simulink model "multi_ca_sim_1"  (R2020a)
settings: Solver=FixedStepAuto  StartTime=0.0  StopTime=23  FixedStep=0.01  MinStep=0.01  RelTol=1e-3
values from neighbouring files (symbols this model uses):
  ar_max = beta^2*omega/gamma/pi*0.999    (= 2.172825)    [SimulationSetup.m]
  beta = pi/tau_r    (= 3.14159265359)    [SimulationSetup.m]
  gamma = tau_r*beta + pi    (= 6.28318530718)    [SimulationSetup.m]
  Gamma = 10    [SimulationSetup.m]
  k = (gamma/beta)^2*(vo_max*psio_max) +0.1    (= 0.235)    [SimulationSetup.m]
  k_1 = 0.2    [SimulationSetup.m]
  k_2 = gamma^2/beta    (= 12.5663706144)    [SimulationSetup.m]
  k_delta = 1    [SimulationSetup.m]
  omega = r + (vr_max + vo_max)*pi/beta +0.1    (= 4.35)    [SimulationSetup.m]
  r = 2.0    (= 2)    [SimulationSetup.m]
  theta_0_1 = 0    [SimulationSetup.m]
  theta_0_2 = 0    [SimulationSetup.m]
  theta_0_3 = 0    [SimulationSetup.m]
  theta_a = pi/4    (= 0.785398163397)    [SimulationSetup.m]
  u_ca_max = 10    [SimulationSetup.m]
  u_tr_max = min(beta,beta^2*omega/(vr_max*gamma))    [SimulationSetup.m]
  vo_max = 0.75    [SimulationSetup.m]
  vr_max = 1.5    [SimulationSetup.m]
  vr_min = 1.0    (= 1)    [SimulationSetup.m]
  x_F_0_1 = -6    [SimulationSetup.m]
  x_F_0_2 = -4    [SimulationSetup.m]
  x_F_0_3 = -5    [SimulationSetup.m]
  y_F_0_1 = 0    [SimulationSetup.m]
  y_F_0_2 = -2    [SimulationSetup.m]
  y_F_0_3 = -4    [SimulationSetup.m]
libraries: cstblocks x3, dspmathops x3
(part 2 of 2)

== matlab function multi_ca_sim_1/MATLAB Function1 ==
  data: rho output; pos_vr input; lambda output; pos_obs input; psi_r input; psi_o input; vo input; vr input; dot_lambda output
function [rho, lambda, dot_lambda] = fcn(pos_vr, pos_obs, psi_r, psi_o, vo, vr)

lambda_vector = pos_obs-pos_vr;
rho = norm(lambda_vector,2);
lambda = atan2(lambda_vector(2), lambda_vector(1) );
dot_lambda = 1/rho*(vo*sin(psi_o - lambda) - vr*sin(psi_r - lambda));

== matlab function multi_ca_sim_1/vehicle2/MATLAB Function ==
  data: u input; y output; tan output
function [y,tan] = fcn(u)
theta = u/(1.5*1.5*4*pi);
y = [cos(theta) -sin(theta); sin(theta) cos(theta)]*[1.5*1.5*4*pi; 0];%*[5+6*pi*sin(pi/4)-6*pi*sin(1.2*pi/4)-0.5 15+6*pi*cos(pi/4)-6*pi*cos(1.2*pi/4)]';
tan = [-y(2); y(1)];

== matlab function multi_ca_sim_1/vehicle2/MATLAB Function1 ==
  data: u input; y output
function y = fcn(u)
theta = u/(1.5*1.5*4*pi);
y = [cos(theta) -sin(theta); sin(theta) cos(theta)]*[1.5*1.5*4*pi; 0];%*[5+6*pi*sin(pi/4)-6*pi*sin(1.2*pi/4)-0.5 15+6*pi*cos(pi/4)-6*pi*cos(1.2*pi/4)]';

== matlab function multi_ca_sim_1/vehicle2/vehicle 1 ==
  data: speed_profile output; speed_target output; v_d_xi output; kappa output; t input; xi input; xi_dot input
function [speed_profile, speed_target, v_d_xi, kappa] = fcn(t,xi,xi_dot)
% vd=1.5;
% psi_d = t/pi/4 - pi/4;
% x_dot = 1.5*cos(psi_d);
% y_dot = 1.5*sin(psi_d);

%trajectory and speed profile
% x_dot = 1*1.5*cos(t/pi/4 - 1.2*pi/4);
% y_dot = 0.9*1.5*sin(t/pi/4 - 1.2*pi/4);
speed_profile = 1.5*1.5;

%v_d(xi)
v_d_xi=1.5*1.5;
% v_d_xi=sqrt((0.9*1.5*cos(xi/pi/4 - 1.2*pi/4))^2+(0.9*1.5*sin(xi/pi/4 - 1.2*pi/4))^2);

%speed of target
speed_target = xi_dot*1.5*1.5;

%culvature
r=1.5*1.5*4*pi;
kappa=1/r;

== matlab function multi_ca_sim_1/Time coordination/MATLAB Function5 ==
  data: xi input; Laplacian input; chi input; xi_dot output; chi_dot output
function [xi_dot, chi_dot] = fcn(xi, Laplacian, chi)
k_P=1;
k_I=0.8571; %0.95;
xi_dot=-k_P*Laplacian*xi+[1; chi(1)+0.6; chi(2)-0.2];
chi_dot=-k_I*[0 1 0; 0 0 1]*Laplacian*xi;

== matlab function multi_ca_sim_1/Subsystem/Subsystem5/Subsystem/MATLAB Function ==
  data: theta input; y output; delta input
function y = fcn(theta,delta)
if abs(theta-delta) <= 10^(-7)
    y=cos(theta);
else 
    y=(sin(theta)-sin(delta))/(theta-delta);
end

== matlab function multi_ca_sim_1/MATLAB Function2 ==
  data: tau output; rho input; loom output; rho_dot input; x4 output
function [tau, loom, x4] = fcn(rho, rho_dot)

loom = min(rho_dot/rho, 0);
if loom > -0.0001
    tau = 1000;
else
    tau = -1/loom;
end

x4 = 1/rho;

== matlab function multi_ca_sim_1/CA controller 1 ==
  data: u output; x1 input; x2 input; x3 input; x5 input; k input; r input; vr input; vo_max input; beta input; gamma input; omega input; ar input; x5 output; x2 output; x3 output; y output; alpha_1 output; alpha_2 output
function [u, x5, x2, x3,y, alpha_1, alpha_2]  = fcn(x1, x2 ,x3, x5, k, r, vr, vo_max,beta, gamma,omega, ar)


x6 = vr;

delta_t = ( pi - abs(wrapToPi_custom(x5-x2)))/(beta);

alpha_2 = -2*beta*omega*x1/(x6+vo_max);
alpha_1 = (k*x1^2 +  x6*max(0,-x3*sin(x5-x2)) -min(0, -ar*cos(x5-x2)) ) /(r + (x6 + vo_max )*delta_t);

 u =  sign_custom(wrapToPi_custom(x5-x2))*(gamma^2/beta*(x1^2  +alpha_1 ) +  alpha_2) + x3  ;
y = sign_custom(wrapToPi_custom(x5-x2));

if x1 >= 0
    u=0;
end

function y = sign_custom(x)

if x >= 0
    y = 1;
else
    y = -1;
end

function lambda = wrapTo2Pi_custom(lambda)
%wrapTo2Pi Wrap angle in radians to [0 2*pi]
%
%   lambdaWrapped = wrapTo2Pi(LAMBDA) wraps angles in LAMBDA, in radians,
%   to the interval [0 2*pi] such that zero maps to zero and 2*pi maps
%   to 2*pi. (In general, positive multiples of 2*pi map to 2*pi and
%   negative multiples of 2*pi map to zero.)
%
%   See also wrapToPi, wrapTo180, wrapTo360.

% Copyright 2007-2008 The MathWorks, Inc.

positiveInput = (lambda > 0);
lambda = mod(lambda, 2*pi);
lambda((lambda == 0) & positiveInput) = 2*pi;

function lambda = wrapToPi_custom(lambda)
%wrapToPi Wrap angle in radians to [-pi pi]
%
%   lambdaWrapped = wrapToPi(LAMBDA) wraps angles in LAMBDA, in radians,
%   to the interval [-pi pi] such that pi maps to pi and -pi maps to
%   -pi.  (In general, odd, positive multiples of pi map to pi and odd,
%   negative multiples of pi map to -pi.)
%
%   See also wrapTo2Pi, wrapTo180, wrapTo360.

% Copyright 2007-2008 The MathWorks, Inc.

q = (lambda < -pi) | (pi < lambda);
lambda(q) = wrapTo2Pi_custom(lambda(q) + pi) - pi;

== matlab function multi_ca_sim_1/Subsystem/MATLAB Function ==
  data: signal input; out output; bound1 input; bound2 input
function out = saturate(signal,bound1,bound2)
out = min(max(bound1,signal),bound2);

== matlab function multi_ca_sim_1/Time coordination/MATLAB Function3 ==
  settings: updateMethod=DISCRETE
  data: t input; y output
function y = fcn(t)

% if rem(u1,exprnd(1))==0
%     y=randi(3);
% %     if rand < 0.3
% %         y=8;
% %     else
% %         y=randi(7);
% %     end
% else
%     y=u2;

% t=u1;

rng('default')

T=[0 exprnd(1,1,60)];
i=randi(10,1,60);

% for j=1:9
%     if t>=sum(T(1:j)) && t<=sum(T(1:j+1))
%         y=i(j);
%     end
% end

        
        
if t>=sum(T(1:1)) && t<=sum(T(1:2))
    y=i(1);
elseif t>=sum(T(1:2)) && t<=sum(T(1:3))
    y=i(2);
elseif t>=sum(T(1:3)) && t<=sum(T(1:4))
    y=i(3);
elseif t>=sum(T(1:4)) && t<=sum(T(1:5))
    y=i(4);
elseif t>=sum(T(1:5)) && t<=sum(T(1:6))
    y=i(5); 
elseif t>=sum(T(1:6)) && t<=sum(T(1:7))
    y=i(6);
elseif t>=sum(T(1:7)) && t<=sum(T(1:8))
    y=i(7);
elseif t>=sum(T(1:8)) && t<=sum(T(1:9))
    y=i(8);
elseif t>=sum(T(1:9)) && t<=sum(T(1:10))
    y=i(9);
elseif t>=sum(T(1:10)) && t<=sum(T(1:11))
    y=i(10);
elseif t>=sum(T(1:11)) && t<=sum(T(1:12))
    y=i(11);
elseif t>=sum(T(1:12)) && t<=sum(T(1:13))
    y=i(12);
elseif t>=sum(T(1:13)) && t<=sum(T(1:14))
    y=i(13);
elseif t>=sum(T(1:14)) && t<=sum(T(1:15))
    y=i(14);
elseif t>=sum(T(1:15)) && t<=sum(T(1:16))
    y=i(15);
elseif t>=sum(T(1:16)) && t<=sum(T(1:17))
    y=i(16);
elseif t>=sum(T(1:17)) && t<=sum(T(1:18))
    y=i(17);
elseif t>=sum(T(1:18)) && t<=sum(T(1:19))
    y=i(18);
elseif t>=sum(T(1:19)) && t<=sum(T(1:20))
    y=i(19);
elseif t>=sum(T(1:20)) && t<=sum(T(1:21))
    y=i(20);
elseif t>=sum(T(1:21)) && t<=sum(T(1:22))
    y=i(21);
elseif t>=sum(T(1:22)) && t<=sum(T(1:23))
    y=i(22);
elseif t>=sum(T(1:23)) && t<=sum(T(1:24))
    y=i(23);
elseif t>=sum(T(1:24)) && t<=sum(T(1:25))
    y=i(24);
elseif t>=sum(T(1:25)) && t<=sum(T(1:26))
    y=i(25);
elseif t>=sum(T(1:26)) && t<=sum(T(1:27))
    y=i(26);
elseif t>=sum(T(1:27)) && t<=sum(T(1:28))
    y=i(27);
elseif t>=sum(T(1:28)) && t<=sum(T(1:29))
    y=i(28);
elseif t>=sum(T(1:29)) && t<=sum(T(1:30))
    y=i(29);
elseif t>=sum(T(1:30)) && t<=sum(T(1:31))
    y=i(30);
    elseif t>=sum(T(1:31)) && t<=sum(T(1:32))
    y=i(31);
    elseif t>=sum(T(1:32)) && t<=sum(T(1:33))
    y=i(32);
    elseif t>=sum(T(1:33)) && t<=sum(T(1:34))
    y=i(33);
    elseif t>=sum(T(1:34)) && t<=sum(T(1:35))
    y=i(34);
    elseif t>=sum(T(1:35)) && t<=sum(T(1:36))
    y=i(35);
    elseif t>=sum(T(1:36)) && t<=sum(T(1:37))
    y=i(36);
    elseif t>=sum(T(1:37)) && t<=sum(T(1:38))
    y=i(37);
    elseif t>=sum(T(1:38)) && t<=sum(T(1:39))
    y=i(38);
    elseif t>=sum(T(1:39)) && t<=sum(T(1:40))
    y=i(39);
    elseif t>=sum(T(1:40)) && t<=sum(T(1:41))
    y=i(40);
    elseif t>=sum(T(1:41)) && t<=sum(T(1:42))
    y=i(41);
    elseif t>=sum(T(1:42)) && t<=sum(T(1:43))
    y=i(42);
    elseif t>=sum(T(1:43)) && t<=sum(T(1:44))
    y=i(43);
    elseif t>=sum(T(1:44)) && t<=sum(T(1:45))
    y=i(44);
    elseif t>=sum(T(1:45)) && t<=sum(T(1:46))
    y=i(45);
    elseif t>=sum(T(1:46)) && t<=sum(T(1:47))
    y=i(46);
    elseif t>=sum(T(1:47)) && t<=sum(T(1:48))
    y=i(47);
    elseif t>=sum(T(1:48)) && t<=sum(T(1:49))
    y=i(48);
    elseif t>=sum(T(1:49)) && t<=sum(T(1:50))
    y=i(49);
    elseif t>=sum(T(1:50)) && t<=sum(T(1:51))
    y=i(50);
    elseif t>=sum(T(1:51)) && t<=sum(T(1:52))
    y=i(51);
    elseif t>=sum(T(1:52)) && t<=sum(T(1:53))
    y=i(52);
    elseif t>=sum(T(1:53)) && t<=sum(T(1:54))
    y=i(53);
    elseif t>=sum(T(1:54)) && t<=sum(T(1:55))
    y=i(54);
    elseif t>=sum(T(1:55)) && t<=sum(T(1:56))
    y=i(55);
    elseif t>=sum(T(1:56)) && t<=sum(T(1:57))
    y=i(56);
    elseif t>=sum(T(1:57)) && t<=sum(T(1:58))
    y=i(57);
    elseif t>=sum(T(1:58)) && t<=sum(T(1:59))
    y=i(58);
    elseif t>=sum(T(1:59)) && t<=sum(T(1:60))
    y=i(59);
    elseif t>=sum(T(1:60)) && t<=sum(T(1:61))
    y=i(60);
else
    y=0;
end



        


end
